simulink model "AKF"  (R2023a)
settings: Solver=VariableStepAuto  StartTime=0.0  StopTime=10.0  RelTol=1e-3
settings Model: Creator=belov  LastModifiedBy=belov

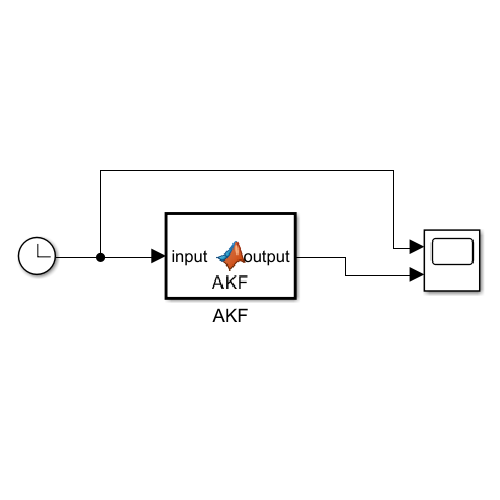
[thumbnail: Simulink's stored preview of the top-level diagram]
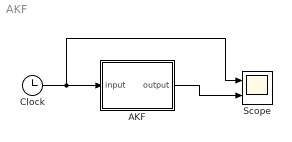
== system AKF ==
  AKF : MATLAB Function  TreatAsAtomicUnit=on
  Clock : Clock
  Scope : Scope  NumInputPorts=2
  wires:
  Clock/1 -> Scope/1, AKF/1(input)
  AKF/1(output) -> Scope/2

== matlab function AKF/AKF ==
  data: input input; output output
function output = AKF(input)
persistent x_last_last P_last_last q_last Q_last r_last R_last;
if(isempty(x_last_last))
    x_last_last = 0;
end
if(isempty(P_last_last))
    P_last_last = 0;
end
if(isempty(q_last))
    q_last = 0;
end
if(isempty(Q_last))
    Q_last = 0.1;
end
if(isempty(r_last))
    r_last = 0;
end
if(isempty(R_last))
    R_last = 0.5;
end

A = 1;
B = 1;
C = 1;

x_last_now = A * x_last_last + B * q_last;
P_last_now = A * P_last_last * A' + B * Q_last * B';

K_now = P_last_now * C' * inv(C * P_last_now * C' + R_last);
delta_now = input - C * x_last_now - r_last;
x_now_now = x_last_now + K_now * delta_now;
I = eye(1);
P_now_now = (I - K_now * C) * P_last_now;

persistent t;
if(isempty(t))
    t = 1;
end
dt = 1 / t;

q_last = (1 - dt) * q_last + dt * (x_now_now - A * x_last_last);
Q_last = (1 - dt) * Q_last + dt * (K_now * delta_now * delta_now' * K_now' + P_now_now - A * P_last_last * A');
r_last = (1 - dt) * r_last + dt * (input - C * x_last_now);
R_last = (1 - dt) * R_last + dt * (delta_now * delta_now' - C * P_last_now * C');
t = t + 1;
x_last_last = x_now_now;
P_last_last = P_now_now;
output = x_now_now;
